simulink model "Test_Euler2DCM"  (Simulink 7.5)
settings: Solver=FixedStepDiscrete  StartTime=0.0  StopTime=1  RelTol=1e-3
libraries: aerolibtransform2 x1
settings Model: Creator=Robert  LastModifiedBy=Robert

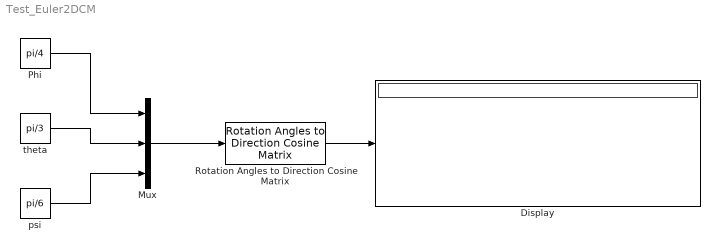
== system Test_Euler2DCM ==
  Display : Display
  Mux : Mux  Inputs=3
  Phi : Constant  Value=pi/4  OutDataTypeMode=single  OutDataType=fixdt(1, 16)  OutScaling=2^0  OutDataTypeStr=single
  Rotation Angles to Direction Cosine Matrix : aerolibtransform2/Rotation Angles to Direction Cosine Matrix  SystemSampleTime=-1  rotationOrder=XYZ
  psi : Constant  Value=pi/6  OutDataTypeMode=single  OutDataType=fixdt(1, 16)  OutScaling=2^0  OutDataTypeStr=single
  theta : Constant  Value=pi/3  OutDataTypeMode=single  OutDataType=fixdt(1, 16)  OutScaling=2^0  OutDataTypeStr=single
  wires:
  Rotation Angles to Direction Cosine Matrix/1 -> Display/1
  Mux/1 -> Rotation Angles to Direction Cosine Matrix/1
  Phi/1 -> Mux/1
  theta/1 -> Mux/2
  psi/1 -> Mux/3
